simulink model "governor_library"  (R2019b)
settings: Solver=VariableStepAuto  StartTime=0.0  StopTime=10.0  RelTol=1e-3
undefined symbols (not defined in the file or in its folder): dyn, govDisable, init, sys
settings Model: Creator=gdudgeon  LastModifiedBy=gdudgeon
settings SFSimCC: CustomCodeUndefinedFunction=UseInterfaceOnly

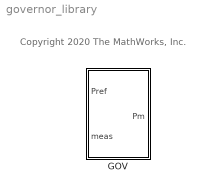
== system governor_library ==
  note: Copyright 2020 The MathWorks, Inc.
  GOV : Subsystem  VariantControlMode=Label  Variant=on  LabelModeActiveChoice=Variant1
      settings: AttributesFormatString=%<BlockChoice>

== system governor_library/GOV ==
  Pref : Inport
  meas : Inport  Port=2
  GGOV1 : Subsystem  VariantControl=Variant1  mask{p=dyn.ggov1_102_GAS, g=sys.GENERATOR(2)}
      mask prompts: p "Parameters"; g "generator"
      mask DialogControl DescGroupVar Prompt: GGOV1
  IEEEG3 : Subsystem  VariantControl=Variant2  mask{p=dyn.ieeeg3_102_HYDRO}
      mask prompts: p "Parameters"
      mask DialogControl DescGroupVar Prompt: IEEEG3
  Pm : Outport  VectorParamsAs1DForOutWhenUnconnected=off

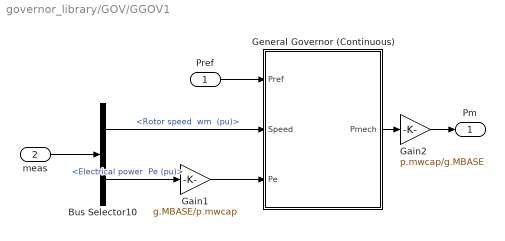
== system governor_library/GOV/GGOV1 ==
  Pref : Inport
  meas : Inport  Port=2
  Bus Selector10 : BusSelector  OutputSignals="Mechanical.Rotor speed  wm  (pu),Mechanical.Electrical power  Pe (pu)"
  Gain1 : Gain  Gain=g.MBASE/p.mwcap
  Gain2 : Gain  Gain=p.mwcap/g.MBASE
  "General Governor (Continuous) " : Subsystem  mask(GGOV1 Governor Model){Tpelec=p.tpelec, Kpgov=p.kpgov, Kigov=p.kigov, Kdgov=p.kdgov, Tdgov=p.tdgov, errvec=[p.minerr p.maxerr], vvec=[p.vmin p.vmax], r=p.r, rselect=Electrical Power, Tact=p.tact, Kturb=p.kturb, wfnl=p.wfnl, Tb=p.tb, Tc=p.tc, Teng=p.teng, Flag=Fuel Flow Proportional to Speed, Tfload=p.tfload, Kpload=p.kpload, Kiload=p.kiload, Ldref=p.ldref, Dm=p.dm, rvec=[p.rclose p.ropen], Kimw=p.kimw, Pmwset=p.pmwset, aset=p.aset, Ka=p.ka, Ta=p.ta, db=p.db, Tsa=p.tsa, Tsb=p.tsb, rlimitvec=[p.rdown p.rup], Tau=1e-4}
      mask prompts: Tpelec "Tpelec, Electrical Power Transducer Time Constant [s]"; Kpgov "Kpgov, Proportional Gain"; Kigov "Kigov, Integral Gain"; Kdgov "Kdgov, Derivative Gain"; Tdgov "Tdgov, Derivative Time Constant [s]"; errvec "[minerr maxerr], Speed Error Limits"; vvec "[vmin vmax], Valve Limits"; r "r, Permanent droop [pu]"; rselect "Feedback for Droop"; Tact "Tact, Actuator Time Constant"; Kturb "Kturb, Turbine Gain"; wfnl "wfnl, No Load Fuel Flow [pu]"; Tb "Tb, Lag Time Constant [s]"; Tc "Tc, Lead Time Constant [s]"; Teng "Teng, Transport Lag for Diesel [s]"; Flag "Fuel Source Characteristic"; Tfload "Tfload, Time Constant [s]"; Kpload "Kpload, Proportional Gain"; Kiload "Kiload, Integral Gain"; Ldref "Ldref, Load Limiter Reference Value [pu]"; Dm "Dm, Speed Sensitivity Coefficient [pu]"; rvec "[rclose ropen], Valve Opening Rates [pu/s]"; Kimw "Kimw, Power Controller Gain"; Pmwset "Pmwset, Power Controller Setpoint [MW]"; aset "aset, Acceleration Limiter Setpoint [pu/s]"; Ka "Ka, Acceleration Limiter Gain"; Ta "Ta, Acceleration Limiter Time Constant [s]"; db "db, Speed Governor Dead Band"; Tsa "Tsa, Temperature Detection Lead [s]"; Tsb "Tsb, Temperature Detection Lag [s]"; rlimitvec "[rdown rup], Load Limit Rates"; Tau "Algebraic Loop Time Constant [s]"
      mask init:
      | minerr = errvec(1);   maxerr = errvec(2);
      | vmin = vvec(1);       vmax = vvec(2);
      | ropen = rvec(2);      rclose = rvec(1);
      | rdown = rlimitvec(1); rup = rlimitvec(2);
      mask TypeOptions rselect: Electrical Power | None - Isochronous Governor | Fuel Valve Stroke - True Stroke | Governor Ouput - Requested Stroke
      mask TypeOptions Flag: Fuel Flow Independent of Speed | Fuel Flow Proportional to Speed
      mask DialogControl Container9 Prompt: Governor
      mask DialogControl Container11 Prompt: Droop
      mask DialogControl Container12 Prompt: Turbine
      mask DialogControl Container13 Prompt: Load Limiter
      mask DialogControl Container16 Prompt: Additional Limits
      mask DialogControl Container8 Prompt: Other
      mask Display:
      | port_label('input',1,'Pref');
      | port_label('input',2,'Speed');
      | port_label('input',3,'Pe');
      | port_label('output',1,'Pmech');
      | 
      | color('blue');disp('GGOV1')
  Pm : Outport  VectorParamsAs1DForOutWhenUnconnected=off
  wires:
  Gain2/1 -> Pm/1
  Gain1/1 -> "General Governor (Continuous) "/3(Pe)
  "General Governor (Continuous) "/1(Pmech) -> Gain2/1
  meas/1 -> Bus Selector10/1
  Pref/1 -> "General Governor (Continuous) "/1(Pref)
  Bus Selector10/2 -> Gain1/1  "<Electrical power  Pe (pu)>"
  Bus Selector10/1 -> "General Governor (Continuous) "/2(Speed)  "<Rotor speed  wm  (pu)>"

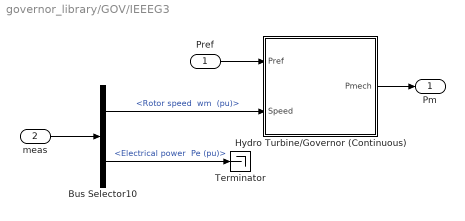
== system governor_library/GOV/IEEEG3 ==
  Pref : Inport
  meas : Inport  Port=2
  Bus Selector10 : BusSelector  OutputSignals="Mechanical.Rotor speed  wm  (pu),Mechanical.Electrical power  Pe (pu)"
  Hydro Turbine/Governor (Continuous) : Subsystem  mask(IEEEG3 Hydro Turbine/Governor Model){Tg=p.tg, Tp=p.tp, Uo=p.uo, Uc=p.uc, Pmax=p.pmax, Pmin=p.pmin, Rperm=p.rperm, Rtemp=p.rtemp, Tr=p.tr, Tw=p.tw, Kturb=p.kturb, Aturb=p.aturb, Bturb=p.bturb, db1=p.db1, eps=p.eps, db2=p.db2, Gv=[p.gv1 p.gv2 p.gv3 p.gv4 p.gv5 p.gv6], Pgv=[p.pgv1 p.pgv2 p.pgv3 p.pgv4 p.pgv5 p.pgv6]}
      mask prompts: Tg "Tg, Gate servo time constant [s]"; Tp "Tp, Pilot servo time constant [s]"; Uo "Uo, Maximum gate opening rate [pu/sec]"; Uc "Uc, Maximum gate closing rate [pu/s]"; Pmax "Pmax, Max gate opening [pu of mw]"; Pmin "Pmin, Minimum gate opening [pu of mx]"; Rperm "Rperm, Permanent droop [pu]"; Rtemp "Rtemp, Temporary droop [pu]"; Tr "Tr, Dashpot time constant [s]"; Tw "Tw, Water inertia time constant [s]"; Kturb "Kturb, Turbine gain [pu]"; Aturb "Aturb, Turbine numerator"; Bturb "Bturb, Turbine denominator"; db1 "db1, Intentional deadband width, Hz"; eps "eps, Intentional deadband hysteresis, Hz"; db2 "db2, Unintentional deadband [MW]"; Gv "Gv, Nonlinear Gain Points [Gv1 Gv2 Gv3 Gv4 Gv5 Gv6], [pu]"; Pgv "Pgv, Nonlinear Gain Points [Pgv1 Pgv2 Pgv3 Pgv4 Pgv5 Pgv6], [pu]"
      mask DialogControl Container9 Prompt: Gate
      mask DialogControl Container11 Prompt: Droop
      mask DialogControl Container12 Prompt: Turbine
      mask DialogControl Container13 Prompt: Nonlinear Effects
      mask Display:
      | port_label('input',1,'Pref');
      | port_label('input',2,'Speed');
      | port_label('output',1,'Pmech');
      | 
      | color('blue');disp('IEEEG3')
  Terminator : Terminator
  Pm : Outport  VectorParamsAs1DForOutWhenUnconnected=off
  wires:
  Bus Selector10/1 -> Hydro Turbine/Governor (Continuous)/2(Speed)  "<Rotor speed  wm  (pu)>"
  Hydro Turbine/Governor (Continuous)/1(Pmech) -> Pm/1
  Bus Selector10/2 -> Terminator/1  "<Electrical power  Pe (pu)>"
  Pref/1 -> Hydro Turbine/Governor (Continuous)/1(Pref)
  meas/1 -> Bus Selector10/1

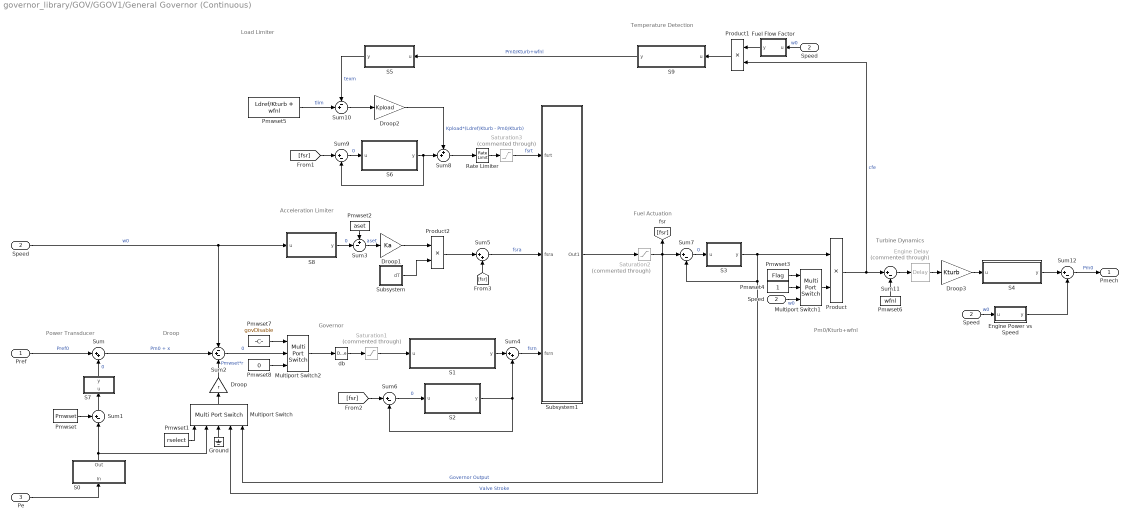
== system governor_library/GOV/GGOV1/General Governor (Continuous)  ==
  note: Pm0/Kturb+wfnl
  note: Load Limiter
  note: Temperature Detection
  note: Turbine Dynamics
  note: Fuel Actuation
  note: Power Transducer
  note: Droop
  note: Governor
  note: Acceleration Limiter
  Pref : Inport
  Speed : Inport  Port=2
  Pe : Inport  Port=3
  " Speed " : InportShadow  Port=2
  Droop : Gain  Gain=r
  Droop1 : Gain  Gain=Ka
  Droop2 : Gain  Gain=Kpload
  Droop3 : Gain  Gain=Kturb
  Engine Delay : TransportDelay  Commented=through  DelayTime=Teng
  Engine Power vs Speed : Subsystem
      mask Display: disp('D_m \times \omega','texmode','on');
  Fuel Flow Factor : Subsystem
      mask Display: disp('\omega^{Dm}','texmode','on');
  Ground : Ground
  Multiport Switch : MultiPortSwitch  Inputs=4
  Multiport Switch1 : MultiPortSwitch  Inputs=2
  Multiport Switch2 : MultiPortSwitch  DataPortOrder=Zero-based contiguous  Inputs=2  zeroidx=on
  Pmwset : Constant  Value=Pmwset
  Pmwset1 : Constant  Value=rselect
  Pmwset2 : Constant  Value=aset
  Pmwset3 : Constant  Value=Flag
  Pmwset4 : Constant
  Pmwset5 : Constant  Value=Ldref/Kturb + wfnl
  Pmwset6 : Constant  Value=wfnl
  Pmwset7 : Constant  Value=govDisable
  Pmwset8 : Constant  Value=0
  Product : Product
  Product1 : Product
  Product2 : Product
  Rate Limiter : RateLimiter  RisingSlewLimit=rup  FallingSlewLimit=rdown  SampleTimeMode=inherited
      settings: AttributesFormatString=|
      | %<RisingSlewLimit>
      | %<FallingSlewLimit>
  S0 : Subsystem
      mask Display: disp('1 / (1 + s T_{pelec})','texmode','on');
  S1 : Subsystem
      mask Display: disp('K_{pgov} + s K_{dgov} / (1 + s T_{dgov})','texmode','on');
  S2 : Subsystem
      mask Display: disp('K_{igov} / (s K_{pgov})','texmode','on');
  S3 : Subsystem
      mask Display: disp('1 / (s T_{act})','texmode','on');
  S4 : Subsystem
      mask Display: disp('(1 + s T_{c}) / (1 + s T_{b})','texmode','on');
  S5 : Subsystem
      mask Display: disp('1 / (1 + s T_{fload})','texmode','on');
  S6 : Subsystem
      mask Display: disp('K_{iload} / (s K_{pload})','texmode','on');
  S7 : Subsystem
      mask Display: disp('K_{imw}/s','texmode','on');
  S8 : Subsystem
      mask Display: disp('s / (1 + s T_a)','texmode','on');
  S9 : Subsystem
      mask Display: disp('(1 + s T_{sa}) / (1 + s T_{sb})','texmode','on');
  Saturation1 : Saturate  Commented=through  UpperLimit=maxerr  LowerLimit=minerr
      settings: AttributesFormatString=|
      | %<UpperLimit>
      | %<LowerLimit>
  Saturation2 : Saturate  Commented=through  UpperLimit=vmax  LowerLimit=vmin
      settings: AttributesFormatString=|
      | %<UpperLimit>
      | %<LowerLimit>
  Saturation3 : Saturate  Commented=through  UpperLimit=1  LowerLimit=-Inf
      settings: AttributesFormatString=|
      | %<UpperLimit>
      | %<LowerLimit>
  "Speed " : InportShadow  Port=2
  "Speed  " : InportShadow  Port=2
  Subsystem : Subsystem
      mask Display: disp('\Delta T','texmode','on');
  Subsystem1 : Subsystem
  Sum : Sum  Inputs=|++
  Sum1 : Sum  Inputs=+-|
  Sum10 : Sum  Inputs=-+|
  Sum{6..7,9,11..12} (5 alike) : Sum  Inputs=|+-
  Sum2 : Sum  Inputs=-+-
  Sum3 : Sum  Inputs=+-|
  Sum4 : Sum  Inputs=|++
  Sum5 : Sum  Inputs=|++
  Sum8 : Sum  Inputs=++|
  db : DeadZone  LowerValue=db  UpperValue=-db  SaturateOnIntegerOverflow=on
  Pmech : Outport  VectorParamsAs1DForOutWhenUnconnected=off
  wires:
  Pmwset8/1 -> Multiport Switch2/3
  Sum2/1 -> Multiport Switch2/2  "0"
  Pmwset7/1 -> Multiport Switch2/1
  Multiport Switch2/1 -> db/1
  Sum4/1 -> Subsystem1/3(fsrn)  "fsrn"
  Sum5/1 -> Subsystem1/2(fsra)  "fsra"
  Saturation3/1 -> Subsystem1/1(fsrt)  "fsrt"
  Multiport Switch1/1 -> Product/2
  Subsystem1/1(Out1) -> Saturation2/1
  Subsystem/1(dT) -> Product2/2
  Product2/1 -> Sum5/1
  Droop1/1 -> Product2/1
  Sum12/1 -> Pmech/1  "Pm0"
  Pref/1 -> Sum/1  "Pref0"
  S7/1(y) -> Sum/2  "0"
  Sum1/1 -> S7/1(u)
  Pmwset/1 -> Sum1/1
  Sum/1 -> Sum2/2  "Pm0 + x"
  Speed/1 -> S8/1(u), Sum2/1  "w0"
  Droop/1 -> Sum2/3  "Pmwset*r"
  S0/1(Out) -> Multiport Switch/2, Sum1/2
  Pe/1 -> S0/1(In)
  Multiport Switch/1 -> Droop/1
  Pmwset1/1 -> Multiport Switch/1
  Ground/1 -> Multiport Switch/3
  S8/1(y) -> Sum3/2  "0"
  Pmwset2/1 -> Sum3/1
  db/1 -> Saturation1/1
  Saturation1/1 -> S1/1(u)
  S1/1(y) -> Sum4/1
  Sum3/1 -> Droop1/1  "aset"
  Saturation2/1 -> Multiport Switch/5, Sum7/1, [fsr]  "Governor Output"
  [fsr] -> Sum6/1
  S2/1(y) -> Sum4/2, Sum6/2
  Sum6/1 -> S2/1(u)  "0"
  [fsr] -> Sum5/2
  Sum7/1 -> S3/1(u)  "0"
  S3/1(y) -> Sum7/2, Multiport Switch/4, Product/1  "Valve Stroke"
  Pmwset3/1 -> Multiport Switch1/1
  Pmwset4/1 -> Multiport Switch1/2
  "Speed "/1 -> Multiport Switch1/3  "w0"
  Product/1 -> Sum11/1, Product1/2  "cfe"
  Rate Limiter/1 -> Saturation3/1
  Sum8/1 -> Rate Limiter/1
  [fsr] -> Sum9/1
  Sum9/1 -> S6/1(u)  "0"
  S6/1(y) -> Sum8/2, Sum9/2
  Droop2/1 -> Sum8/1  "Kpload*(Ldref/Kturb - Pm0/Kturb)"
  Sum10/1 -> Droop2/1
  Pmwset5/1 -> Sum10/2  "tlim"
  S5/1(y) -> Sum10/1  "texm"
  S9/1(y) -> S5/1(u)  "Pm0/Kturb+wfnl"
  Product1/1 -> S9/1(u)
  "Speed  "/1 -> Fuel Flow Factor/1(u)  "w0"
  Fuel Flow Factor/1(y) -> Product1/1
  Pmwset6/1 -> Sum11/2
  Sum11/1 -> Engine Delay/1
  Engine Delay/1 -> Droop3/1
  Droop3/1 -> S4/1(u)
  S4/1(y) -> Sum12/1
  Engine Power vs Speed/1(y) -> Sum12/2
  " Speed "/1 -> Engine Power vs Speed/1(u)  "w0"

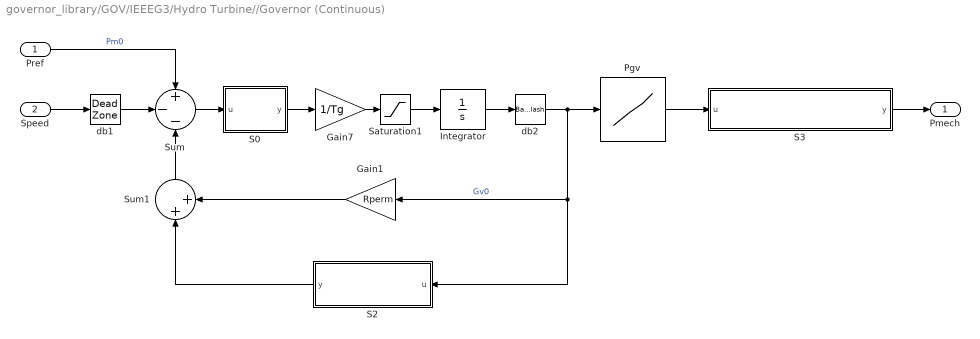
== system governor_library/GOV/IEEEG3/Hydro Turbine//Governor (Continuous) ==
  Pref : Inport
  Speed : Inport  Port=2
  Gain1 : Gain  Gain=Rperm
  Gain7 : Gain  Gain=1/Tg
  Integrator : Integrator  LimitOutput=on  UpperSaturationLimit=Pmax  LowerSaturationLimit=Pmin
      settings: AttributesFormatString=|
      | %<UpperSaturationLimit>
      | %<LowerSaturationLimit>
  Pgv : Lookup_n-D  NumberOfTableDimensions=1  BreakpointsForDimension1=[0 Gv 1]  Table=[0 Pgv 1]  InternalRulePriority=Speed  RndMeth=Simplest  InputSameDT=on
  S0 : Subsystem
      mask Display: disp('1/(1+sTp)')
  S2 : Subsystem
      mask Display: disp('R_{temp} s T_r / (1 + s T_r)','texmode','on');
  S3 : Subsystem
      mask Display: disp('R_{turb} (1 + s A_{turb} T_w) / (1 + s B_{turb} T_w)','texmode','on');
  Saturation1 : Saturate  UpperLimit=Uo  LowerLimit=Uc
      settings: AttributesFormatString=|
      | %<UpperLimit>
      | %<LowerLimit>
  Sum : Sum  Inputs=+--
  Sum1 : Sum  Inputs=|++
  db1 : DeadZone  LowerValue=db1  UpperValue=-db1  SaturateOnIntegerOverflow=on
  db2 : Backlash  BacklashWidth=2*db2  ZeroCross=off
  Pmech : Outport  InitialOutput=0  VectorParamsAs1DForOutWhenUnconnected=off
  wires:
  db2/1 -> Gain1/1, S2/1(u), Pgv/1  "Gv0"
  Pgv/1 -> S3/1(u)
  Sum1/1 -> Sum/3
  Integrator/1 -> db2/1
  S2/1(y) -> Sum1/1
  Sum/1 -> S0/1(u)
  S3/1(y) -> Pmech/1
  Gain1/1 -> Sum1/2
  db1/1 -> Sum/2
  Pref/1 -> Sum/1  "Pm0"
  Speed/1 -> db1/1
  Saturation1/1 -> Integrator/1
  S0/1(y) -> Gain7/1
  Gain7/1 -> Saturation1/1

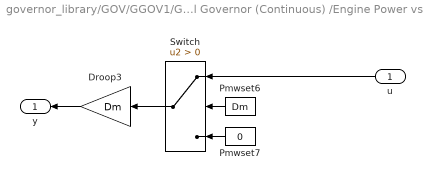
== system governor_library/GOV/GGOV1/General Governor (Continuous) /Engine Power vs Speed ==
  u : Inport
  Droop3 : Gain  Gain=Dm
  Pmwset6 : Constant  Value=Dm
  Pmwset7 : Constant  Value=0
  Switch : Switch  Criteria=u2 > Threshold  ZeroCross=off
  y : Outport  VectorParamsAs1DForOutWhenUnconnected=off
  wires:
  Pmwset6/1 -> Switch/2
  Pmwset7/1 -> Switch/3
  Switch/1 -> Droop3/1
  Droop3/1 -> y/1
  u/1 -> Switch/1

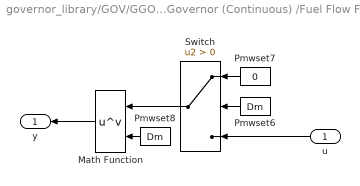
== system governor_library/GOV/GGOV1/General Governor (Continuous) /Fuel Flow Factor ==
  u : Inport
  Math Function : Math  Operator=pow  SaturateOnIntegerOverflow=on
  Pmwset6 : Constant  Value=Dm
  Pmwset7 : Constant  Value=0
  Pmwset8 : Constant  Value=Dm
  Switch : Switch  Criteria=u2 > Threshold  ZeroCross=off
  y : Outport  VectorParamsAs1DForOutWhenUnconnected=off
  wires:
  Pmwset6/1 -> Switch/2
  Switch/1 -> Math Function/1
  Pmwset8/1 -> Math Function/2
  Math Function/1 -> y/1
  u/1 -> Switch/3
  Pmwset7/1 -> Switch/1

== system governor_library/GOV/GGOV1/General Governor (Continuous) /S0 ==
  In : Inport
  1/Tpelec : Gain  Gain=1/Tpelec
  Integrator : Integrator
  Sum : Sum  Inputs=|+-
  Out : Outport  InitialOutput=0  VectorParamsAs1DForOutWhenUnconnected=off
  wires:
  Integrator/1 -> Out/1, Sum/2
  In/1 -> Sum/1
  1/Tpelec/1 -> Integrator/1
  Sum/1 -> 1/Tpelec/1

== system governor_library/GOV/GGOV1/General Governor (Continuous) /S1 ==
  u : Inport
  Droop1 : Gain  Gain=Kpgov
  S1_TF : Subsystem
      mask Display: disp('s K_{dgov} / (1 + s T_{dgov})','texmode','on');
  Sum4 : Sum  Inputs=++|
  y : Outport  InitialOutput=0  VectorParamsAs1DForOutWhenUnconnected=off
  wires:
  u/1 -> S1_TF/1(u), Droop1/1
  Droop1/1 -> Sum4/2
  S1_TF/1(y) -> Sum4/1  "0"
  Sum4/1 -> y/1  "Pm0*Kpgov"

== system governor_library/GOV/GGOV1/General Governor (Continuous) /S2 ==
  u : Inport
  Droop2 : Gain  Gain=Kigov/Kpgov
  Integrator : Integrator
  y : Outport  InitialOutput=0  VectorParamsAs1DForOutWhenUnconnected=off
  wires:
  u/1 -> Droop2/1
  Droop2/1 -> Integrator/1
  Integrator/1 -> y/1

== system governor_library/GOV/GGOV1/General Governor (Continuous) /S3 ==
  u : Inport
  Droop2 : Gain  Gain=1/Tact
  Integrator : Integrator  InitialCondition=1
  Saturation3 : Saturate  Commented=through  UpperLimit=ropen  LowerLimit=rclose
      settings: AttributesFormatString=|
      | %<UpperLimit>
      | %<LowerLimit>
  y : Outport  InitialOutput=0  VectorParamsAs1DForOutWhenUnconnected=off
  wires:
  Integrator/1 -> y/1
  Saturation3/1 -> Integrator/1
  Droop2/1 -> Saturation3/1
  u/1 -> Droop2/1

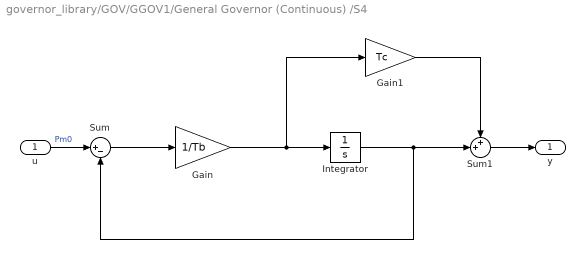
== system governor_library/GOV/GGOV1/General Governor (Continuous) /S4 ==
  u : Inport
  Gain : Gain  Gain=1/Tb
  Gain1 : Gain  Gain=Tc
  Integrator : Integrator  InitialCondition=1
  Sum : Sum  Inputs=|+-
  Sum1 : Sum  Inputs=++|
  y : Outport  InitialOutput=0  VectorParamsAs1DForOutWhenUnconnected=off
  wires:
  Gain1/1 -> Sum1/1
  Integrator/1 -> Sum/2, Sum1/2
  u/1 -> Sum/1  "Pm0"
  Sum/1 -> Gain/1
  Gain/1 -> Gain1/1, Integrator/1
  Sum1/1 -> y/1

== system governor_library/GOV/GGOV1/General Governor (Continuous) /S5 ==
  u : Inport
  1/Tfload : Gain  Gain=1/Tfload
  Integrator : Integrator
  Sum : Sum  Inputs=|+-
  y : Outport  InitialOutput=0  VectorParamsAs1DForOutWhenUnconnected=off
  wires:
  Integrator/1 -> y/1, Sum/2
  u/1 -> Sum/1
  1/Tfload/1 -> Integrator/1
  Sum/1 -> 1/Tfload/1

== system governor_library/GOV/GGOV1/General Governor (Continuous) /S6 ==
  u : Inport
  Droop2 : Gain  Gain=Kiload/Kpload
  Integrator : Integrator
  y : Outport  InitialOutput=0  VectorParamsAs1DForOutWhenUnconnected=off
  wires:
  Integrator/1 -> y/1
  Droop2/1 -> Integrator/1
  u/1 -> Droop2/1

== system governor_library/GOV/GGOV1/General Governor (Continuous) /S7 ==
  u : Inport
  Gain1 : Gain  Gain=Kimw
  Integrator : Integrator  UpperSaturationLimit=1.1*r  LowerSaturationLimit=-1.1*r
      settings: AttributesFormatString=|
      | %<UpperSaturationLimit>
      | %<LowerSaturationLimit>
  y : Outport  InitialOutput=0  VectorParamsAs1DForOutWhenUnconnected=off
  wires:
  Integrator/1 -> y/1
  Gain1/1 -> Integrator/1
  u/1 -> Gain1/1

== system governor_library/GOV/GGOV1/General Governor (Continuous) /S8 ==
  u : Inport
  Gain : Gain  Gain=1/Ta
  Integrator : Integrator
  Sum : Sum  Inputs=|+-
  y : Outport  InitialOutput=0  VectorParamsAs1DForOutWhenUnconnected=off
  wires:
  Integrator/1 -> Sum/2
  Sum/1 -> Gain/1
  u/1 -> Sum/1
  Gain/1 -> y/1, Integrator/1

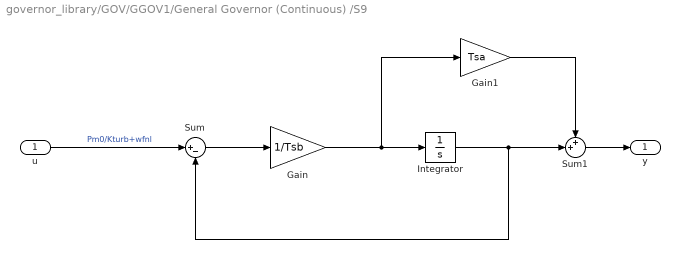
== system governor_library/GOV/GGOV1/General Governor (Continuous) /S9 ==
  u : Inport
  Gain : Gain  Gain=1/Tsb
  Gain1 : Gain  Gain=Tsa
  Integrator : Integrator
  Sum : Sum  Inputs=|+-
  Sum1 : Sum  Inputs=++|
  y : Outport  InitialOutput=0  VectorParamsAs1DForOutWhenUnconnected=off
  wires:
  Sum1/1 -> y/1
  Gain/1 -> Gain1/1, Integrator/1
  Sum/1 -> Gain/1
  u/1 -> Sum/1  "Pm0/Kturb+wfnl"
  Integrator/1 -> Sum1/2, Sum/2
  Gain1/1 -> Sum1/1

== system governor_library/GOV/GGOV1/General Governor (Continuous) /Subsystem ==
  Clock : Clock
  Memory : Memory  InitialCondition=-0.2
  Sum13 : Sum  Inputs=|+-
  dT : Outport  VectorParamsAs1DForOutWhenUnconnected=off
  wires:
  Memory/1 -> Sum13/2
  Clock/1 -> Memory/1, Sum13/1
  Sum13/1 -> dT/1

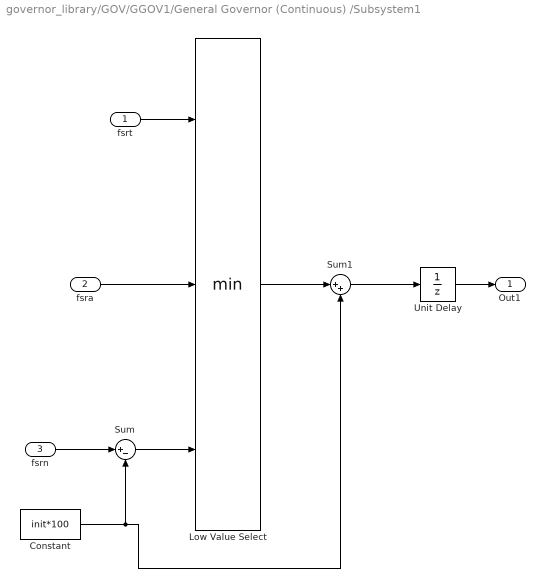
== system governor_library/GOV/GGOV1/General Governor (Continuous) /Subsystem1 ==
  fsrt : Inport
  fsra : Inport  Port=2
  fsrn : Inport  Port=3
  Constant : Constant  Value=init*100
  Low Value Select : MinMax  Inputs=3  ZeroCross=off
  Sum : Sum  Inputs=|+-
  Sum1 : Sum  Inputs=|++
  Unit Delay : UnitDelay  SampleTime=-1  HasFrameUpgradeWarning=on
  Out1 : Outport  VectorParamsAs1DForOutWhenUnconnected=off
  wires:
  Constant/1 -> Sum/2, Sum1/2
  Sum1/1 -> Unit Delay/1
  Low Value Select/1 -> Sum1/1
  Sum/1 -> Low Value Select/3
  fsrn/1 -> Sum/1
  Unit Delay/1 -> Out1/1
  fsrt/1 -> Low Value Select/1
  fsra/1 -> Low Value Select/2

== system governor_library/GOV/IEEEG3/Hydro Turbine//Governor (Continuous)/S0 ==
  u : Inport
  1/Tp : Gain  Gain=1/Tp
  Integrator : Integrator
  Sum : Sum  Inputs=|+-
  y : Outport  VectorParamsAs1DForOutWhenUnconnected=off
  wires:
  Sum/1 -> 1/Tp/1
  1/Tp/1 -> Integrator/1
  u/1 -> Sum/1
  Integrator/1 -> Sum/2, y/1

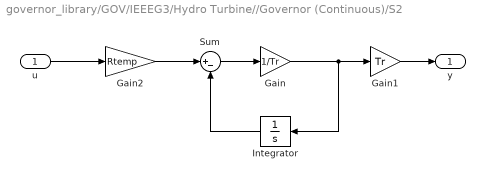
== system governor_library/GOV/IEEEG3/Hydro Turbine//Governor (Continuous)/S2 ==
  u : Inport
  Gain : Gain  Gain=1/Tr
  Gain1 : Gain  Gain=Tr
  Gain2 : Gain  Gain=Rtemp
  Integrator : Integrator
  Sum : Sum  Inputs=|+-
  y : Outport  InitialOutput=0  VectorParamsAs1DForOutWhenUnconnected=off
  wires:
  Gain2/1 -> Sum/1
  u/1 -> Gain2/1
  Sum/1 -> Gain/1
  Gain/1 -> Integrator/1, Gain1/1
  Integrator/1 -> Sum/2
  Gain1/1 -> y/1

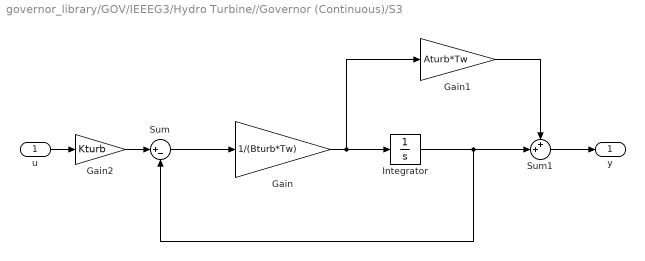
== system governor_library/GOV/IEEEG3/Hydro Turbine//Governor (Continuous)/S3 ==
  u : Inport
  Gain : Gain  Gain=1/(Bturb*Tw)
  Gain1 : Gain  Gain=Aturb*Tw
  Gain2 : Gain  Gain=Kturb
  Integrator : Integrator  InitialCondition=1
  Sum : Sum  Inputs=|+-
  Sum1 : Sum  Inputs=++|
  y : Outport  InitialOutput=0  VectorParamsAs1DForOutWhenUnconnected=off
  wires:
  Gain1/1 -> Sum1/1
  Integrator/1 -> Sum/2, Sum1/2
  Gain2/1 -> Sum/1
  Sum/1 -> Gain/1
  Gain/1 -> Integrator/1, Gain1/1
  Sum1/1 -> y/1
  u/1 -> Gain2/1

== system governor_library/GOV/GGOV1/General Governor (Continuous) /S1/S1_TF ==
  u : Inport
  Gain : Gain  Gain=1/Tdgov
  Gain1 : Gain  Gain=Kdgov
  Integrator : Integrator  InitialCondition=-Pmwset*r
  Sum : Sum  Inputs=|+-
  y : Outport  VectorParamsAs1DForOutWhenUnconnected=off
  wires:
  Gain/1 -> Gain1/1, Integrator/1
  Integrator/1 -> Sum/2
  Sum/1 -> Gain/1
  u/1 -> Sum/1
  Gain1/1 -> y/1
